simulink model "motor_speed_control"  (R2020b)
settings: Solver=VariableStepAuto  StartTime=0.0  StopTime=10.0  RelTol=1e-3
model workspace (MAT data in the model file):
  Ke = Simulink.Parameter
  Ke.Value = 1
  Ke.DataType = 'auto'
  Ke.Dimensions = [1 1]
  Ki = Simulink.Parameter
  Ki.Value = 1
  Ki.DataType = 'auto'
  Ki.Dimensions = [1 1]
libraries: simulink x1, pid_lib x1
settings Model: Creator=shivanshu shukla  LastModifiedBy=shivanshu shukla

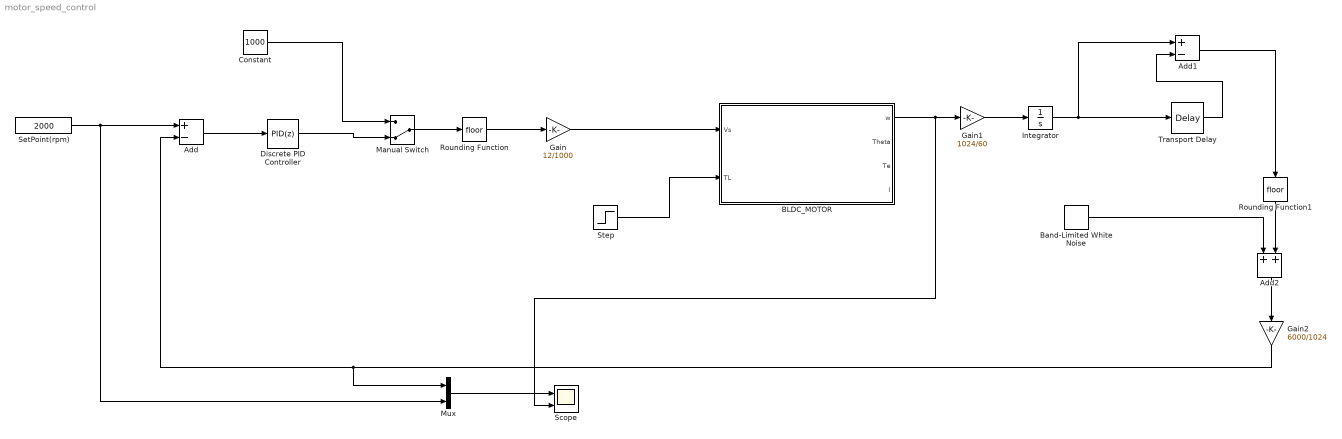
== system motor_speed_control ==
  Add : Sum  Inputs=+-
  Add1 : Sum  Inputs=+-
  Add2 : Sum
  BLDC_MOTOR : Subsystem
  Band-Limited White Noise : simulink/Sources/Band-Limited White Noise  Cov=[0.1]  Ts=0.1  seed=[23341]
  Constant : Constant  Value=1000
  Discrete PID Controller : pid_lib/PID Controller  Controller=PID  Form=Parallel  TimeDomain=Discrete-time  UseExternalTs=off  SampleTime=-1  IntegratorMethod=Forward Euler  FilterMethod=Forward Euler  ControllerParametersSource=internal  P=1  I=1  D=0  UseFilter=on  N=100  TunerSelectOption=Transfer Function Based (PID Tuner App)  InitialConditionSource=internal  InitialConditionForIntegrator=0  InitialConditionForFilter=0  DifferentiatorICPrevScaledInput=0  ExternalReset=none  TrackingMode=off  Kt=1  LimitOutput=off  SatLimitsSource=internal  UpperSaturationLimit=inf  LowerSaturationLimit=-inf  LinearizeAsGain=off  AntiWindupMode=none  Kb=1  POutMin=[]  POutMax=[]  IOutMin=[]  IOutMax=[]  DOutMin=[]  DOutMax=[]  NOutMin=[]  NOutMax=[]  SumOutMin=[]  SumOutMax=[]  SaturationOutMin=[]  SaturationOutMax=[]  PParamMin=[]  PParamMax=[]  IParamMin=[]  IParamMax=[]  DParamMin=[]  DParamMax=[]  NParamMin=[]  NParamMax=[]  KbParamMin=[]  KbParamMax=[]  KtParamMin=[]  KtParamMax=[]  KbOutMin=[]  KbOutMax=[]  KtOutMin=[]  KtOutMax=[]  IntegratorOutMin=[]  IntegratorOutMax=[]  FilterOutMin=[]  FilterOutMax=[]  SumI1OutMin=[]  SumI1OutMax=[]  SumI2OutMin=[]  SumI2OutMax=[]  SumI3OutMin=[]  SumI3OutMax=[]  SumI4OutMin=[]  SumI4OutMax=[]  SumDOutMin=[]  SumDOutMax=[]  DifferentiatorOutMin=[]  DifferentiatorOutMax=[]  FilterDiffOutCoefMin=[]  FilterDiffOutCoefMax=[]  ReciprocalOutMin=[]  ReciprocalOutMax=[]  SumDenOutMin=[]  SumDenOutMax=[]  SumNumOutMin=[]  SumNumOutMax=[]  DivideOutMin=[]  DivideOutMax=[]  UdiffTsProdOutMin=[]  UdiffTsProdOutMax=[]  NTsProdOutMin=[]  NTsProdOutMax=[]  UintegralTsProdOutMin=[]  UintegralTsProdOutMax=[]  UngainTsProdOutMin=[]  UngainTsProdOutMax=[]  IntegratorContinuousStateAttributes=''  IntegratorStateMustResolveToSignalObject=off  IntegratorRTWStateStorageClass=Auto  FilterContinuousStateAttributes=''  FilterStateMustResolveToSignalObject=off  FilterRTWStateStorageClass=Auto  ParallelPVariant=InternalParameters  IdealPVariant=Disabled  IVariant=InternalParameters  DVariant=InternalParameters  IntegratorVariant=Discrete  SatVariant=Disabled  AWVariant=Passthrough  PCopyVariant=Disabled  TRVariant=Disabled  FdbkBlocksVariant=Forward  IdealPFdbkVariant=Disabled  SatFdbkVariant=Disabled  DerivativeFilterVariant=ForwardEulerFilter  NVariant=InternalParameters  NCopyVariant=Disabled  FilterICVariant=InternalICsFilter  IntegratorICVariant=InternalICs  ExternalResetVariant=Disabled  TRSumVariant=Passthrough  SumFdbkVariant=Disabled  SumVariant=Sum_PID  TsampFilterVariant=InternalTs  TsampNgainVariant=Passthrough  TsampIntegralVariant=Passthrough  ExternalSaturationOutDataTypeStr=Inherit: Same as second input
  Gain : Gain  Gain=12/1000
  Gain1 : Gain  Gain=1024/60
  Gain2 : Gain  Gain=6000/1024
  Integrator : Integrator
  Manual Switch : ManualSwitch  CurrentSetting=0
  Mux : Mux  Inputs=2
  Rounding Function : Rounding
  Rounding Function1 : Rounding
  Scope : Scope  NumInputPorts=2
  SetPoint(rpm) : Constant  Value=2000
  Step : Step  SampleTime=0
  Transport Delay : TransportDelay
  wires:
  Rounding Function/1 -> Gain/1
  Gain/1 -> BLDC_MOTOR/1(Vs)
  Manual Switch/1 -> Rounding Function/1
  Constant/1 -> Manual Switch/1
  Add/1 -> Discrete PID Controller/1
  Discrete PID Controller/1 -> Manual Switch/2
  SetPoint(rpm)/1 -> Add/1, Mux/2
  BLDC_MOTOR/1(w) -> Gain1/1, Scope/2
  Gain1/1 -> Integrator/1
  Integrator/1 -> Transport Delay/1, Add1/1
  Transport Delay/1 -> Add1/2
  Add1/1 -> Rounding Function1/1
  Rounding Function1/1 -> Add2/2
  Band-Limited White Noise/1 -> Add2/1
  Add2/1 -> Gain2/1
  Gain2/1 -> Mux/1, Add/2
  Mux/1 -> Scope/1
  Step/1 -> BLDC_MOTOR/2(TL)

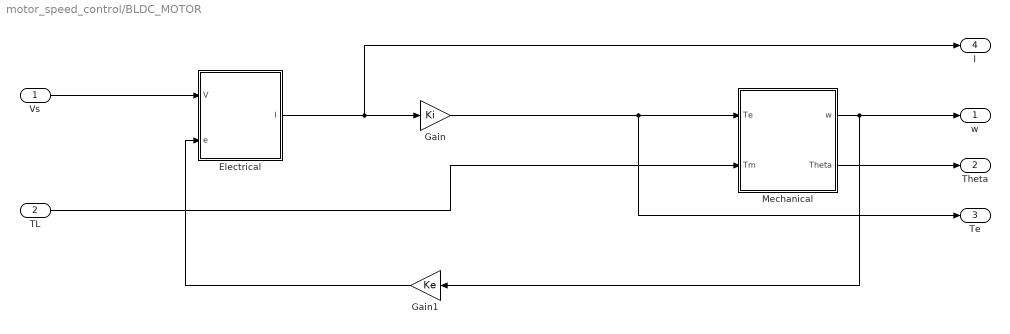
== system motor_speed_control/BLDC_MOTOR ==
  Vs : Inport
  TL : Inport  Port=2
  Electrical : Subsystem
  Gain : Gain  Gain=Ki
  Gain1 : Gain  Gain=Ke
  Mechanical : Subsystem
  w : Outport
  Theta : Outport  Port=2
  Te : Outport  Port=3
  I : Outport  Port=4
  wires:
  Mechanical/2(Theta) -> Theta/1
  Mechanical/1(w) -> w/1, Gain1/1
  Electrical/1(I) -> I/1, Gain/1
  Gain/1 -> Te/1, Mechanical/1(Te)
  TL/1 -> Mechanical/2(Tm)
  Gain1/1 -> Electrical/2(e)
  Vs/1 -> Electrical/1(V)

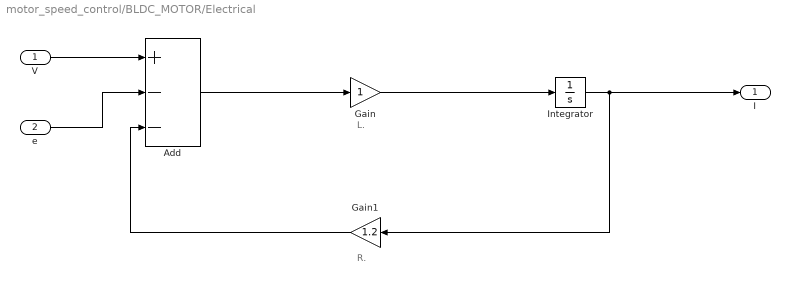
== system motor_speed_control/BLDC_MOTOR/Electrical ==
  note: L.
  note: R.
  V : Inport
  e : Inport  Port=2
  Add : Sum  Inputs=+--
  Gain : Gain
  Gain1 : Gain  Gain=1.2
  Integrator : Integrator
  I : Outport
  wires:
  Gain1/1 -> Add/3
  Integrator/1 -> I/1, Gain1/1
  Gain/1 -> Integrator/1
  e/1 -> Add/2
  V/1 -> Add/1
  Add/1 -> Gain/1

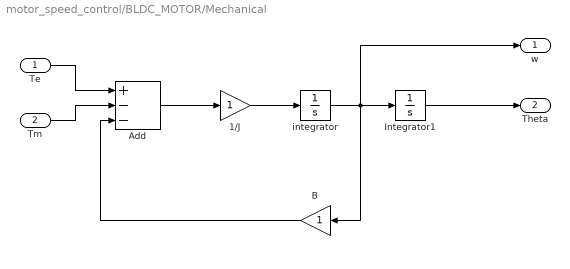
== system motor_speed_control/BLDC_MOTOR/Mechanical ==
  Te : Inport
  Tm : Inport  Port=2
  1/J : Gain
  Add : Sum  Inputs=+--
  B : Gain
  Integrator1 : Integrator
  integrator : Integrator
  w : Outport
  Theta : Outport  Port=2
  wires:
  Integrator1/1 -> Theta/1
  1/J/1 -> integrator/1
  integrator/1 -> w/1, B/1, Integrator1/1
  Add/1 -> 1/J/1
  Tm/1 -> Add/2
  B/1 -> Add/3
  Te/1 -> Add/1
